simulink model "FailSafe_Simulation"  (R2023b)
settings: Solver=VariableStepAuto  StartTime=0.0  StopTime=10.0  RelTol=1e-3
undefined symbols (not defined in the file): DiscIntNeverNeededParam
settings Model: Creator=Amir  LastModifiedBy=vahed
settings SolverCC: AlgebraicLoopSolver=TrustRegion
settings DataIOCC: ReturnWorkspaceOutputs=off
settings DebuggingCC: UnconnectedInputMsg=warning  UnconnectedOutputMsg=warning  UnconnectedLineMsg=warning  ArithmeticOperatorsInVariantConditions=warning
settings ModelReferenceCC: EnableRefExpFcnMdlSchedulingChecks=on
settings SFSimCC: CustomCodeUndefinedFunction=UseInterfaceOnly

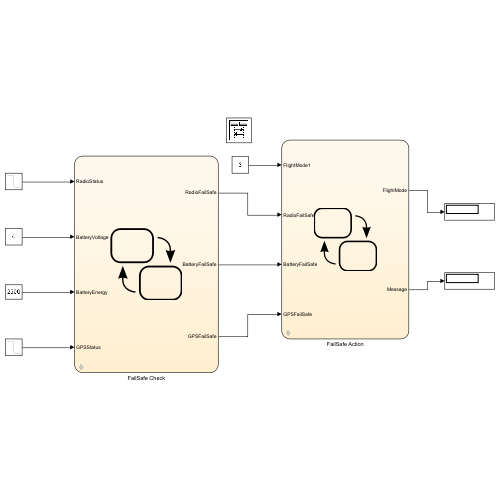
[thumbnail: Simulink's stored preview of the top-level diagram]
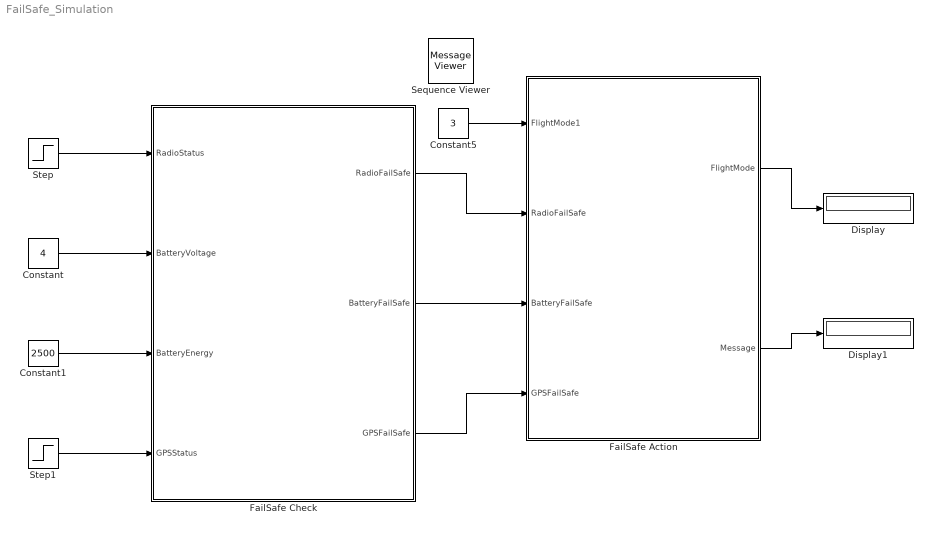
== system FailSafe_Simulation ==
  Constant : Constant  Value=4
  Constant1 : Constant  Value=2500
  Constant5 : Constant  Value=3
  Display : Display
  Display1 : Display
  FailSafe Action : Stateflow chart  TreatAsAtomicUnit=on  mask(FailSafe FlightModes){RadioChoice=RTL, BatteryChoice=Disarm, GCSChoice=RTL, GPSChoice=Land, EKFChoice=Land, Min_H_Parach=150}
      mask prompts: RadioChoice "Flight Mode for Radio FailSafe"; BatteryChoice "Flight Mode for Battery FailSafe"; GCSChoice "Flight Mode for GCS FailSafe"; GPSChoice "Flight Mode for GPS FailSafe"; EKFChoice "Flight Mode for EKF FailSafe"; Min_H_Parach "Min Height to Use Parachute"
  FailSafe Check : Stateflow chart  TreatAsAtomicUnit=on  mask(FailSafe Parameters){FailVoltage=5, FailCapacity=2000, EKFThershold=0.6, RollThershold=55}
      mask prompts: FailVoltage "Voltage Thershold(V)"; FailCapacity "Capacity Thershold(mA.h)"; EKFThershold "EKF Variance Thershold"; RollThershold "Roll Angle Thershold(Degree)"
  Sequence Viewer : MessageViewer
  Step : Step  Before=1  After=0  SampleTime=0
  Step1 : Step  Before=1  After=0  SampleTime=0
  wires:
  FailSafe Action/1(FlightMode) -> Display/1
  Constant5/1 -> FailSafe Action/1(FlightMode1)
  FailSafe Check/1(RadioFailSafe) -> FailSafe Action/2(RadioFailSafe)
  FailSafe Action/2(Message) -> Display1/1
  Step1/1 -> FailSafe Check/4(GPSStatus)
  Constant1/1 -> FailSafe Check/3(BatteryEnergy)
  Step/1 -> FailSafe Check/1(RadioStatus)
  Constant/1 -> FailSafe Check/2(BatteryVoltage)
  FailSafe Check/2(BatteryFailSafe) -> FailSafe Action/3(BatteryFailSafe)
  FailSafe Check/3(GPSFailSafe) -> FailSafe Action/4(GPSFailSafe)

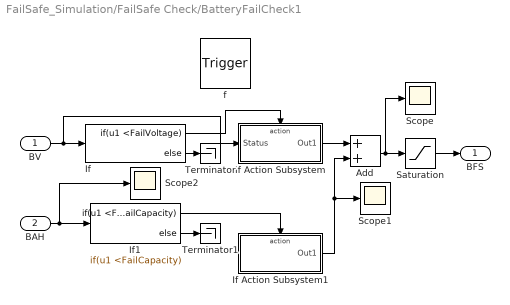
== system FailSafe_Simulation/FailSafe Check/BatteryFailCheck1 ==
  BV : Inport  OutDataTypeStr=double  PortDimensions=1
  BAH : Inport  Port=2  OutDataTypeStr=double  PortDimensions=1
  f : TriggerPort  TriggerType=function-call  VariantControl=(inherit)
      settings: CopyFcn=Stateflow.SLINSF.SimulinkMan.removeBlockPreDeleteFcn  PreDeleteFcn=Stateflow.SLINSF.SimulinkMan.unsafePredeleteFcn
  Add : Sum
  If : If  IfExpression=u1 <FailVoltage
  If Action Subsystem : Subsystem  TreatAsAtomicUnit=on
  If Action Subsystem1 : Subsystem  TreatAsAtomicUnit=on
  If1 : If  IfExpression=u1 <FailCapacity
  Saturation : Saturate  UpperLimit=1  LowerLimit=0
  Scope : Scope
  Scope1 : Scope
  Scope2 : Scope
  Terminator : Terminator
  Terminator1 : Terminator
  BFS : Outport  VectorParamsAs1DForOutWhenUnconnected=off
  wires:
  BV/1 -> If Action Subsystem/1(Status), If/1
  If/1 -> If Action Subsystem/Action
  If Action Subsystem/1(Out1) -> Add/1
  If/2 -> Terminator/1
  BAH/1 -> Scope2/1, If1/1
  If1/1 -> If Action Subsystem1/Action
  If Action Subsystem1/1(Out1) -> Scope1/1, Add/2
  Add/1 -> Saturation/1, Scope/1
  If1/2 -> Terminator1/1
  Saturation/1 -> BFS/1

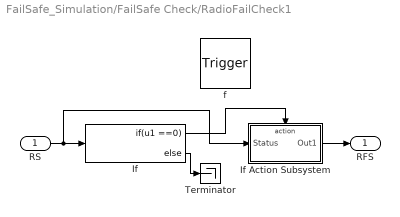
== system FailSafe_Simulation/FailSafe Check/RadioFailCheck1 ==
  RS : Inport  OutDataTypeStr=double  PortDimensions=1
  f : TriggerPort  TriggerType=function-call  VariantControl=(inherit)
      settings: CopyFcn=Stateflow.SLINSF.SimulinkMan.removeBlockPreDeleteFcn  PreDeleteFcn=Stateflow.SLINSF.SimulinkMan.unsafePredeleteFcn
  If : If  IfExpression=u1 ==0
  If Action Subsystem : Subsystem  TreatAsAtomicUnit=on
  Terminator : Terminator
  RFS : Outport  VectorParamsAs1DForOutWhenUnconnected=off
  wires:
  RS/1 -> If Action Subsystem/1(Status), If/1
  If/1 -> If Action Subsystem/Action
  If Action Subsystem/1(Out1) -> RFS/1
  If/2 -> Terminator/1

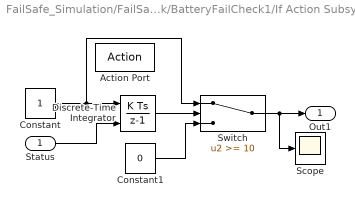
== system FailSafe_Simulation/FailSafe Check/BatteryFailCheck1/If Action Subsystem ==
  Status : Inport
  Action Port : ActionPort  InitializeStates=reset  ActionPortLabel=if { }
  Constant : Constant
  Constant1 : Constant  Value=0
  Discrete-Time Integrator : DiscreteIntegrator  gainval=1  ExternalReset=rising  SampleTime=-1  ICPrevOutput=DiscIntNeverNeededParam  ICPrevScaledInput=DiscIntNeverNeededParam
  Scope : Scope
  Switch : Switch  Threshold=10  SaturateOnIntegerOverflow=off  InputSameDT=off
  Out1 : Outport  VectorParamsAs1DForOutWhenUnconnected=off
  wires:
  Constant/1 -> Switch/1, Discrete-Time Integrator/1
  Status/1 -> Discrete-Time Integrator/2
  Discrete-Time Integrator/1 -> Switch/2
  Constant1/1 -> Switch/3
  Switch/1 -> Out1/1, Scope/1

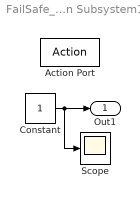
== system FailSafe_Simulation/FailSafe Check/BatteryFailCheck1/If Action Subsystem1 ==
  Action Port : ActionPort  InitializeStates=reset  ActionPortLabel=if { }
  Constant : Constant
  Scope : Scope
  Out1 : Outport  InitialOutput=[0]  VectorParamsAs1DForOutWhenUnconnected=off
  wires:
  Constant/1 -> Scope/1, Out1/1

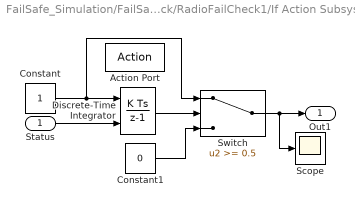
== system FailSafe_Simulation/FailSafe Check/RadioFailCheck1/If Action Subsystem ==
  Status : Inport
  Action Port : ActionPort  InitializeStates=reset  ActionPortLabel=if { }
  Constant : Constant
  Constant1 : Constant  Value=0
  Discrete-Time Integrator : DiscreteIntegrator  gainval=1  ExternalReset=rising  SampleTime=-1  ICPrevOutput=DiscIntNeverNeededParam  ICPrevScaledInput=DiscIntNeverNeededParam
  Scope : Scope
  Switch : Switch  Threshold=0.5  SaturateOnIntegerOverflow=off  InputSameDT=off
  Out1 : Outport  VectorParamsAs1DForOutWhenUnconnected=off
  wires:
  Constant/1 -> Switch/1, Discrete-Time Integrator/1
  Status/1 -> Discrete-Time Integrator/2
  Discrete-Time Integrator/1 -> Switch/2
  Constant1/1 -> Switch/3
  Switch/1 -> Out1/1, Scope/1

== stateflow chart FailSafe_Simulation/FailSafe Action ==
  state Radio [parallel]
    settings: executionOrder=1
    state RadioAction
      if RadioFailSafe
      if FlightMode1 ==1
      FlightMode=FlightMode1
      else
      switch RadioChoice
      case 2
      FlightMode=2
      case 1
      FlightMode=1
      case 3
      FlightMode=3
      end
      end
      Message=1;
      end
    (default) -> RadioAction
  state Battery [parallel]
    settings: executionOrder=2
    state BatteryAction
      if BatteryFailSafe
      if FlightMode1 ==1 || FlightMode1 ==2
      FlightMode=FlightMode1
      else
      switch BatteryChoice
      case 2
      FlightMode=2
      case 1
      FlightMode=1
      case 3
      FlightMode=0
      end
      end
      Message=2;
      end
    (default) -> BatteryAction
  state GPS [parallel]
    settings: executionOrder=3
    state GPSAction
      if GPSFailSafe
      if FlightMode1 ==4
      FlightMode=FlightMode1
      else
      switch GPSChoice
      case 2
      FlightMode=4
      case 1
      FlightMode=1
      case 3
      FlightMode=5
      end
      end
      Message=4;
      end
    (default) -> GPSAction
  data: FlightMode1 input; RadioFailSafe input; BatteryFailSafe input; GPSFailSafe input; FlightMode output; Message output; RadioChoice parameter; BatteryChoice parameter; GCSChoice parameter; GPSChoice parameter; EKFChoice parameter; Min_H_Parach parameter

== stateflow chart FailSafe_Simulation/FailSafe Check ==
  state FailSafeCheck
    state FailSafeCheck
      RadioFailSafe=RadioFailCheck(RadioStatus);
      BatteryFailSafe=BatteryFailCheck(BatteryVoltage,BatteryEnergy);
      GPSFailSafe=GPSFailCheck(GPSStatus);
    (default) -> FailSafeCheck.FailSafeCheck
  state RFS=RadioFailCheck(RS) [function]
    (default) -> (junction 15)
    (junction 15) -> (junction 16) [order 1] : [RS==0]
    (junction 15) -> (junction 17) [order 2] : {RFS=0;}
    (junction 16) -> (junction 18) : {RFS=1;}
    (junction 18) -> (junction 17)
    (junction 17) -> (junction 19)
  state GPSFS=GPSFailCheck(GPSS) [function]
    (default) -> (junction 76)
    (junction 76) -> (junction 77) [order 1] : [GPSS==0]
    (junction 76) -> (junction 78) [order 2] : {GPSFS=0;}
    (junction 77) -> (junction 79) : {GPSFS=1;}
    (junction 79) -> (junction 78)
    (junction 78) -> (junction 80)
  state BFS=BatteryFailCheck(BV,BAH) [function]
    (default) -> (junction 32)
    (junction 32) -> (junction 50) [order 2] : [BAH<=FailCapacity&&BAH~=0]
    (junction 32) -> (junction 33) [order 1] : [BV<=FailVoltage]
    (junction 50) -> (junction 48) : {BFS=1;}
    (junction 32) -> (junction 34) [order 3] : {BFS=0;}
    (junction 33) -> (junction 35) : {BFS=1;}
    (junction 48) -> (junction 34)
    (junction 35) -> (junction 34)
    (junction 34) -> (junction 36)
  state RFS=RadioFailCheck1(RS) [function]
  state BFS=BatteryFailCheck1(BV,BAH) [function]
  data: RS function_input; RFS function_output; GPSS function_input; GPSFS function_output; BV function_input; BFS function_output; BAH function_input; FailVoltage parameter; FailCapacity parameter; RS function_input double size=1; RFS function_output; BV function_input double size=1; BFS function_output; BAH function_input double size=1; RadioStatus input; RadioFailSafe output; BatteryVoltage input; BatteryEnergy input; BatteryFailSafe output; GPSStatus input; GPSFailSafe output
